simulink model "sampleModel7125_pp"  (R2018a)
settings: Solver=VariableStepAuto  StartTime=0.0  StopTime=10.0  RelTol=1e-3
undefined symbols (not defined in the file or in its folder): DiscIntNeverNeededParam
libraries: simulink x93
(part 1 of 2)
settings Model: Creator=cyfuzz  LastModifiedBy=ishaf
settings CodeAppCC: StateflowObjectComments=on

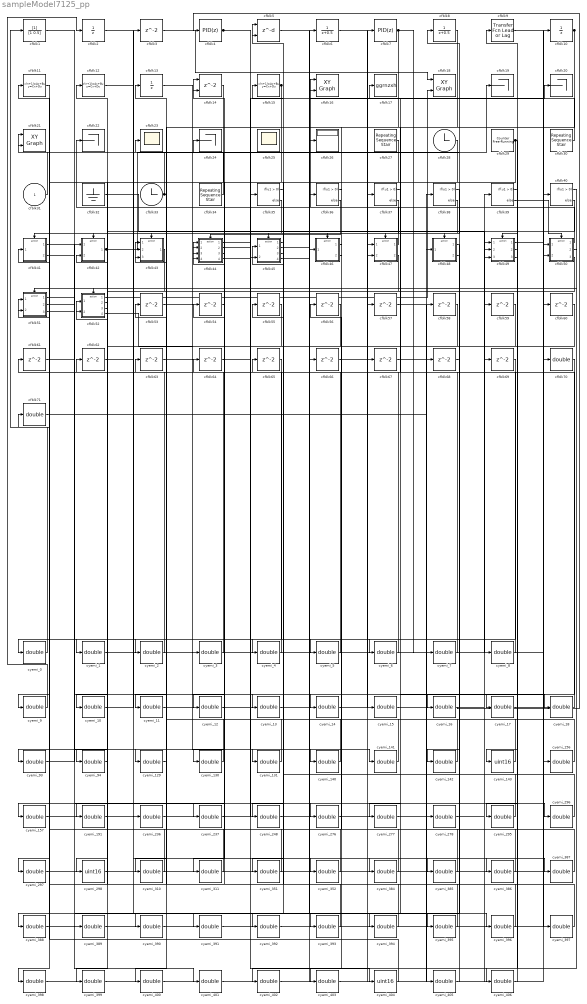
== system sampleModel7125_pp ==
  cfblk31 : Inport
  cfblk1 : DiscreteFilter  SampleTime=1
  cfblk10 : UnitDelay
  cfblk11 : DiscreteStateSpace
  cfblk12 : DiscreteStateSpace
  cfblk13 : UnitDelay
  cfblk14 : Delay  ShowEnablePort=on  SampleTime=1
      settings: InputPortMap=u0,e6
  cfblk15 : DiscreteStateSpace
  cfblk16 : simulink/Sinks/XY Graph  xmin=-1  xmax=1  ymin=-1  ymax=1  st=-1
  cfblk17 : ToWorkspace  VariableName=ggrnzxh  SaveFormat=Timeseries  SampleTime=-1
  cfblk18 : simulink/Sinks/XY Graph  xmin=-1  xmax=1  ymin=-1  ymax=1  st=-1
  cfblk{19..20,22,24} (4 alike) : Terminator
  cfblk2 : UnitDelay
  cfblk21 : simulink/Sinks/XY Graph  xmin=-1  xmax=1  ymin=-1  ymax=1  st=-1
  cfblk23 : Scope
  cfblk25 : Scope
      settings: Floating=on
  cfblk26 : Display
  cfblk27 : simulink/Sources/Repeating Sequence Stair  OutValues=[3 1 4 2 1].'  tsamp=1  OutMin=[]  OutMax=[]  OutDataTypeStr=double  OutputDataTypeScalingMode=double  OutDataType=fixdt(0,8)  ConRadixGroup=Best Precision: Vector-wise  OutScaling=2^-12
  cfblk28 : Clock
  cfblk29 : simulink/Sources/Counter Free-Running  NumBits=16  tsamp=1
  cfblk{3,53..69} (18 alike) : Delay  SampleTime=1
  cfblk30 : simulink/Sources/Repeating Sequence Stair  OutValues=[3 1 4 2 1].'  tsamp=1  OutMin=[]  OutMax=[]  OutDataTypeStr=double  OutputDataTypeScalingMode=double  OutDataType=fixdt(0,8)  ConRadixGroup=Best Precision: Vector-wise  OutScaling=2^-12
  cfblk32 : Ground
  cfblk33 : Clock
  cfblk34 : simulink/Sources/Repeating Sequence Stair  OutValues=[3 1 4 2 1].'  tsamp=1  OutMin=[]  OutMax=[]  OutDataTypeStr=double  OutputDataTypeScalingMode=double  OutDataType=fixdt(0,8)  ConRadixGroup=Best Precision: Vector-wise  OutScaling=2^-12
  cfblk{35..40} (6 alike) : If  SampleTime=1
  cfblk4 : simulink/Continuous/PID Controller  Controller=PID  TimeDomain=Discrete-time  SampleTime=1  IntegratorMethod=Forward Euler  FilterMethod=Forward Euler  Form=Parallel  UseFilter=on  ControllerParametersSource=internal  P=1  I=1  D=0  N=100  InitialConditionSource=internal  InitialConditionForIntegrator=0  InitialConditionForFilter=0  ExternalReset=none  LimitOutput=off  UpperSaturationLimit=inf  LowerSaturationLimit=-inf  LinearizeAsGain=off  AntiWindupMode=none  Kb=1  TrackingMode=off  Kt=1  PParamMin=[]  PParamMax=[]  IParamMin=[]  IParamMax=[]  DParamMin=[]  DParamMax=[]  NParamMin=[]  NParamMax=[]  KbParamMin=[]  KbParamMax=[]  KtParamMin=[]  KtParamMax=[]  POutMin=[]  POutMax=[]  IOutMin=[]  IOutMax=[]  DOutMin=[]  DOutMax=[]  NOutMin=[]  NOutMax=[]  KbOutMin=[]  KbOutMax=[]  KtOutMin=[]  KtOutMax=[]  IntegratorOutMin=[]  IntegratorOutMax=[]  FilterOutMin=[]  FilterOutMax=[]  SumOutMin=[]  SumOutMax=[]  SumI1OutMin=[]  SumI1OutMax=[]  SumI2OutMin=[]  SumI2OutMax=[]  SumI3OutMin=[]  SumI3OutMax=[]  SumDOutMin=[]  SumDOutMax=[]  SaturationOutMin=[]  SaturationOutMax=[]  IntegratorContinuousStateAttributes=''  IntegratorStateMustResolveToSignalObject=off  IntegratorRTWStateStorageClass=Auto  FilterContinuousStateAttributes=''  FilterStateMustResolveToSignalObject=off  FilterRTWStateStorageClass=Auto  DifferentiatorICPrevScaledInput=0  DifferentiatorOutMin=[]  DifferentiatorOutMax=[]  FilterDiffOutCoefMin=[]  FilterDiffOutCoefMax=[]  SumDenOutMin=[]  SumDenOutMax=[]  SumNumOutMin=[]  SumNumOutMax=[]  ReciprocalOutMin=[]  ReciprocalOutMax=[]  DivideOutMin=[]  DivideOutMax=[]  TunerSelectOption=Transfer Function Based (PID Tuner App)
  cfblk41 : Subsystem  TreatAsAtomicUnit=on
  cfblk42 : Subsystem  TreatAsAtomicUnit=on
  cfblk43 : Subsystem  TreatAsAtomicUnit=on
  cfblk44 : Subsystem  TreatAsAtomicUnit=on
  cfblk45 : Subsystem  TreatAsAtomicUnit=on
  cfblk46 : Subsystem  TreatAsAtomicUnit=on
  cfblk47 : Subsystem  TreatAsAtomicUnit=on
  cfblk48 : Subsystem  TreatAsAtomicUnit=on
  cfblk49 : Subsystem  TreatAsAtomicUnit=on
  cfblk5 : Delay  DelayLengthSource=Input port  SampleTime=1
      settings: InputPortMap=u0,p1
  cfblk50 : Subsystem  TreatAsAtomicUnit=on
  cfblk51 : Subsystem  TreatAsAtomicUnit=on
  cfblk52 : Subsystem  TreatAsAtomicUnit=on
  cfblk6 : DiscreteTransferFcn  SampleTime=1
  cfblk7 : simulink/Continuous/PID Controller  Controller=PID  TimeDomain=Discrete-time  SampleTime=1  IntegratorMethod=Forward Euler  FilterMethod=Forward Euler  Form=Parallel  UseFilter=on  ControllerParametersSource=internal  P=1  I=1  D=0  N=100  InitialConditionSource=internal  InitialConditionForIntegrator=0  InitialConditionForFilter=0  ExternalReset=none  LimitOutput=off  UpperSaturationLimit=inf  LowerSaturationLimit=-inf  LinearizeAsGain=off  AntiWindupMode=none  Kb=1  TrackingMode=off  Kt=1  PParamMin=[]  PParamMax=[]  IParamMin=[]  IParamMax=[]  DParamMin=[]  DParamMax=[]  NParamMin=[]  NParamMax=[]  KbParamMin=[]  KbParamMax=[]  KtParamMin=[]  KtParamMax=[]  POutMin=[]  POutMax=[]  IOutMin=[]  IOutMax=[]  DOutMin=[]  DOutMax=[]  NOutMin=[]  NOutMax=[]  KbOutMin=[]  KbOutMax=[]  KtOutMin=[]  KtOutMax=[]  IntegratorOutMin=[]  IntegratorOutMax=[]  FilterOutMin=[]  FilterOutMax=[]  SumOutMin=[]  SumOutMax=[]  SumI1OutMin=[]  SumI1OutMax=[]  SumI2OutMin=[]  SumI2OutMax=[]  SumI3OutMin=[]  SumI3OutMax=[]  SumDOutMin=[]  SumDOutMax=[]  SaturationOutMin=[]  SaturationOutMax=[]  IntegratorContinuousStateAttributes=''  IntegratorStateMustResolveToSignalObject=off  IntegratorRTWStateStorageClass=Auto  FilterContinuousStateAttributes=''  FilterStateMustResolveToSignalObject=off  FilterRTWStateStorageClass=Auto  DifferentiatorICPrevScaledInput=0  DifferentiatorOutMin=[]  DifferentiatorOutMax=[]  FilterDiffOutCoefMin=[]  FilterDiffOutCoefMax=[]  SumDenOutMin=[]  SumDenOutMax=[]  SumNumOutMin=[]  SumNumOutMax=[]  ReciprocalOutMin=[]  ReciprocalOutMax=[]  DivideOutMin=[]  DivideOutMax=[]  TunerSelectOption=Transfer Function Based (PID Tuner App)
  cfblk70 : DataTypeConversion  OutDataTypeStr=double
  cfblk71 : DataTypeConversion  OutDataTypeStr=double
  cfblk8 : DiscreteTransferFcn  SampleTime=1
  cfblk9 : simulink/Discrete/Transfer Fcn Lead or Lag  PoleZ=0.95  ZeroZ=0.75  ICPrevOutput=0.0  ICPrevInput=0.0  DoSatur=off
      settings: SourceProductName=Simulink  SourceProductBaseCode=SL
  cyemi_{0..18,93..94,129..131,140..142,156..157,191,236..237,248,276..278,295..297,310..311,351..352,384..403,405..406} (65 alike) : DataTypeConversion  OutDataTypeStr=double
  cyemi_143 : DataTypeConversion  OutDataTypeStr=uint16
  cyemi_298 : DataTypeConversion  OutDataTypeStr=uint16
  cyemi_404 : DataTypeConversion  OutDataTypeStr=uint16
  wires:
  cfblk34/1 -> cfblk24/1
  cfblk3/1 -> cfblk18/1
  cfblk15/1 -> cyemi_398/1, cyemi_399/1
  cfblk47/1(cfblk2) -> cfblk16/1
  cfblk30/1 -> cfblk16/2
  cfblk7/1 -> cyemi_7/1, cyemi_400/1
  cfblk33/1 -> cfblk21/2, cyemi_2/1
  cfblk31/1 -> cfblk21/1
  cfblk29/1 -> cyemi_143/1, cyemi_298/1
  cfblk52/1(cfblk2) -> cfblk18/2
  cfblk10/1 -> cyemi_5/1, cyemi_394/1
  cfblk48/2(cfblk7) -> cfblk23/1
  cfblk42/1(cfblk2) -> cfblk19/1, cyemi_384/1
  cfblk50/1(cfblk2) -> cfblk22/1
  cfblk4/1 -> cyemi_385/1, cyemi_386/1
  cfblk45/4(cfblk16) -> cfblk26/1
  cfblk44/2(cfblk15) -> cfblk20/1
  cfblk35/1 -> cfblk41/Action
  cfblk35/2 -> cfblk42/Action
  cfblk36/1 -> cfblk43/Action
  cfblk36/2 -> cfblk44/Action
  cfblk37/1 -> cfblk45/Action
  cfblk37/2 -> cfblk46/Action
  cfblk38/1 -> cfblk47/Action
  cfblk38/2 -> cfblk48/Action
  cfblk39/1 -> cfblk49/Action
  cfblk39/2 -> cfblk50/Action
  cfblk40/1 -> cfblk51/Action
  cfblk40/2 -> cfblk52/Action
  cyemi_0/1 -> cfblk1/1
  cfblk11/1 -> cyemi_0/1
  cyemi_1/1 -> cfblk10/1
  cfblk52/2(cfblk8) -> cyemi_1/1
  cyemi_2/1 -> cfblk11/1
  cyemi_3/1 -> cfblk12/1
  cfblk52/4(cfblk10) -> cyemi_3/1
  cyemi_4/1 -> cfblk13/1
  cfblk45/3(cfblk15) -> cyemi_4/1
  cyemi_5/1 -> cfblk14/1
  cyemi_6/1 -> cfblk14/2
  cfblk58/1 -> cyemi_6/1
  cyemi_7/1 -> cfblk15/1
  cyemi_8/1 -> cfblk17/1
  cfblk32/1 -> cyemi_8/1
  cyemi_9/1 -> cfblk2/1
  cfblk69/1 -> cyemi_9/1
  cyemi_10/1 -> cfblk3/1
  cfblk52/3(cfblk9) -> cyemi_10/1
  cyemi_11/1 -> cfblk35/1
  cfblk14/1 -> cyemi_11/1
  cyemi_12/1 -> cfblk36/1
  cfblk28/1 -> cyemi_12/1
  cyemi_13/1 -> cfblk37/1
  cfblk51/3(cfblk16) -> cyemi_13/1
  cyemi_14/1 -> cfblk38/1
  cfblk64/1 -> cyemi_14/1
  cyemi_15/1 -> cfblk39/1
  cfblk66/1 -> cyemi_15/1
  cyemi_16/1 -> cfblk4/1
  cfblk6/1 -> cyemi_16/1
  cyemi_17/1 -> cfblk40/1
  cfblk57/1 -> cyemi_17/1
  cyemi_18/1 -> cfblk41/1(cfblk1)
  cfblk13/1 -> cyemi_18/1
  cyemi_93/1 -> cfblk42/1(cfblk1)
  cfblk50/3(cfblk14) -> cyemi_93/1
  cyemi_94/1 -> cfblk42/2(cfblk13)
  cfblk43/1(cfblk2) -> cyemi_94/1
  cyemi_129/1 -> cfblk43/1(cfblk1)
  cfblk1/1 -> cyemi_129/1
  cyemi_130/1 -> cfblk43/2(cfblk8)
  cfblk54/1 -> cyemi_130/1
  cyemi_131/1 -> cfblk43/3(cfblk9)
  cfblk53/1 -> cyemi_131/1
  cyemi_140/1 -> cfblk44/1(cfblk1)
  cfblk51/1(cfblk2) -> cyemi_140/1
  cyemi_141/1 -> cfblk44/2(cfblk12)
  cfblk63/1 -> cyemi_141/1
  cyemi_142/1 -> cfblk44/3(cfblk13)
  cfblk68/1 -> cyemi_142/1
  cyemi_143/1 -> cfblk44/4(cfblk14)
  cyemi_156/1 -> cfblk45/1(cfblk1)
  cfblk49/1(cfblk2) -> cyemi_156/1
  cyemi_157/1 -> cfblk45/2(cfblk13)
  cfblk44/3(cfblk16) -> cyemi_157/1
  cyemi_191/1 -> cfblk46/1(cfblk1)
  cfblk59/1 -> cyemi_191/1
  cyemi_236/1 -> cfblk47/1(cfblk1)
  cfblk2/1 -> cyemi_236/1
  cyemi_237/1 -> cfblk47/2(cfblk12)
  cfblk55/1 -> cyemi_237/1
  cyemi_248/1 -> cfblk48/1(cfblk1)
  cfblk56/1 -> cyemi_248/1
  cyemi_276/1 -> cfblk49/1(cfblk1)
  cfblk61/1 -> cyemi_276/1
  cyemi_277/1 -> cfblk49/2(cfblk14)
  cfblk70/1 -> cyemi_277/1
  cyemi_278/1 -> cfblk49/3(cfblk15)
  cfblk67/1 -> cyemi_278/1
  cyemi_295/1 -> cfblk5/1
  cfblk49/2(cfblk16) -> cyemi_295/1
  cyemi_296/1 -> cfblk5/2
  cfblk44/4(cfblk17) -> cyemi_296/1
  cyemi_297/1 -> cfblk50/1(cfblk1)
  cfblk65/1 -> cyemi_297/1
  cyemi_298/1 -> cfblk50/2(cfblk12)
  cyemi_310/1 -> cfblk51/1(cfblk1)
  cfblk47/2(cfblk13) -> cyemi_310/1
  cyemi_311/1 -> cfblk51/2(cfblk14)
  cfblk60/1 -> cyemi_311/1
  cyemi_351/1 -> cfblk52/1(cfblk1)
  cfblk27/1 -> cyemi_351/1
  cyemi_352/1 -> cfblk52/2(cfblk7)
  cfblk62/1 -> cyemi_352/1
  cyemi_384/1 -> cfblk53/1
  cyemi_385/1 -> cfblk54/1
  cyemi_386/1 -> cfblk55/1
  cyemi_387/1 -> cfblk56/1
  cfblk45/2(cfblk14) -> cyemi_387/1
  cyemi_388/1 -> cfblk57/1
  cfblk48/1(cfblk2) -> cyemi_388/1
  cyemi_389/1 -> cfblk58/1
  cfblk41/1(cfblk2) -> cyemi_389/1
  cyemi_390/1 -> cfblk59/1
  cfblk41/2(cfblk14) -> cyemi_390/1
  cyemi_391/1 -> cfblk6/1
  cfblk45/1(cfblk2) -> cyemi_391/1
  cyemi_392/1 -> cfblk60/1
  cfblk46/1(cfblk2) -> cyemi_392/1
  cyemi_393/1 -> cfblk61/1
  cfblk46/2(cfblk16) -> cyemi_393/1
  cyemi_394/1 -> cfblk62/1
  cyemi_395/1 -> cfblk63/1
  cfblk12/1 -> cyemi_395/1
  cyemi_396/1 -> cfblk64/1
  cfblk5/1 -> cyemi_396/1
  cyemi_397/1 -> cfblk65/1
  cfblk9/1 -> cyemi_397/1
  cyemi_398/1 -> cfblk66/1
  cyemi_399/1 -> cfblk67/1
  cyemi_400/1 -> cfblk68/1
  cyemi_401/1 -> cfblk69/1
  cfblk51/2(cfblk15) -> cyemi_401/1
  cyemi_402/1 -> cfblk7/1
  cfblk50/2(cfblk13) -> cyemi_402/1
  cyemi_403/1 -> cfblk70/1
  cfblk8/1 -> cyemi_403/1
  cyemi_404/1 -> cfblk71/1
  cfblk44/1(cfblk2) -> cyemi_404/1
  cyemi_405/1 -> cfblk8/1
  cfblk71/1 -> cyemi_405/1
  cyemi_406/1 -> cfblk9/1
  cfblk49/3(cfblk17) -> cyemi_406/1

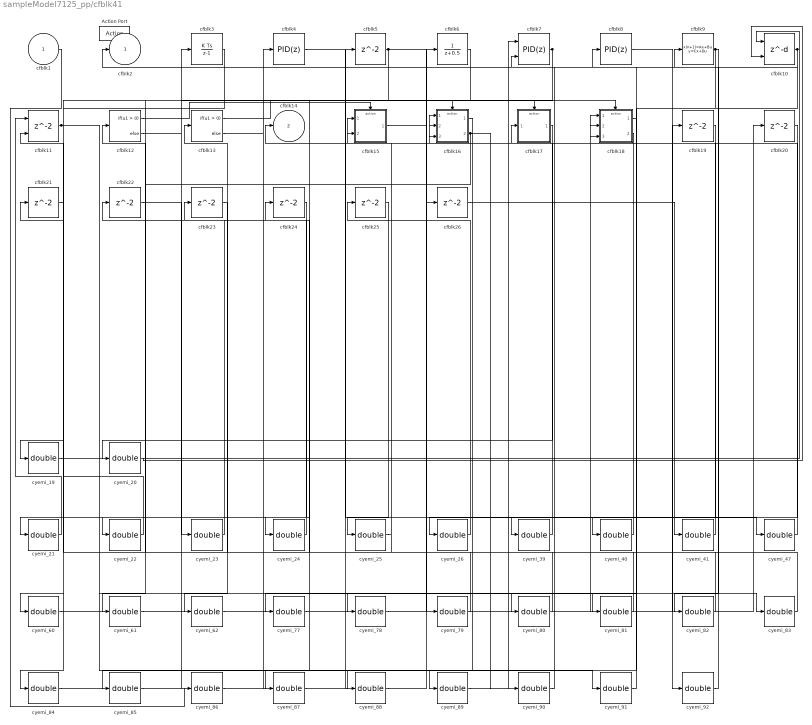
== system sampleModel7125_pp/cfblk41 ==
  cfblk1 : Inport
  Action Port : ActionPort  ActionType=then
  cfblk10 : Delay  DelayLengthSource=Input port
      settings: InputPortMap=u0,p1
  cfblk11 : Delay  ShowEnablePort=on
      settings: InputPortMap=u0,e6
  cfblk12 : If  SampleTime=1
  cfblk13 : If  SampleTime=1
  cfblk15 : Subsystem  TreatAsAtomicUnit=on
  cfblk16 : Subsystem  TreatAsAtomicUnit=on
  cfblk17 : Subsystem  TreatAsAtomicUnit=on
  cfblk18 : Subsystem  TreatAsAtomicUnit=on
  cfblk{5,19..26} (9 alike) : Delay
  cfblk3 : DiscreteIntegrator  SampleTime=-1  OutDataTypeStr=double  ICPrevOutput=DiscIntNeverNeededParam  ICPrevScaledInput=DiscIntNeverNeededParam
  cfblk4 : simulink/Continuous/PID Controller  Controller=PID  TimeDomain=Discrete-time  SampleTime=-1  IntegratorMethod=Forward Euler  FilterMethod=Forward Euler  Form=Parallel  UseFilter=on  ControllerParametersSource=internal  P=1  I=1  D=0  N=100  InitialConditionSource=internal  InitialConditionForIntegrator=0  InitialConditionForFilter=0  ExternalReset=none  LimitOutput=off  UpperSaturationLimit=inf  LowerSaturationLimit=-inf  LinearizeAsGain=off  AntiWindupMode=none  Kb=1  TrackingMode=off  Kt=1  PParamMin=[]  PParamMax=[]  IParamMin=[]  IParamMax=[]  DParamMin=[]  DParamMax=[]  NParamMin=[]  NParamMax=[]  KbParamMin=[]  KbParamMax=[]  KtParamMin=[]  KtParamMax=[]  POutMin=[]  POutMax=[]  IOutMin=[]  IOutMax=[]  DOutMin=[]  DOutMax=[]  NOutMin=[]  NOutMax=[]  KbOutMin=[]  KbOutMax=[]  KtOutMin=[]  KtOutMax=[]  IntegratorOutMin=[]  IntegratorOutMax=[]  FilterOutMin=[]  FilterOutMax=[]  SumOutMin=[]  SumOutMax=[]  SumI1OutMin=[]  SumI1OutMax=[]  SumI2OutMin=[]  SumI2OutMax=[]  SumI3OutMin=[]  SumI3OutMax=[]  SumDOutMin=[]  SumDOutMax=[]  SaturationOutMin=[]  SaturationOutMax=[]  IntegratorContinuousStateAttributes=''  IntegratorStateMustResolveToSignalObject=off  IntegratorRTWStateStorageClass=Auto  FilterContinuousStateAttributes=''  FilterStateMustResolveToSignalObject=off  FilterRTWStateStorageClass=Auto  DifferentiatorICPrevScaledInput=0  DifferentiatorOutMin=[]  DifferentiatorOutMax=[]  FilterDiffOutCoefMin=[]  FilterDiffOutCoefMax=[]  SumDenOutMin=[]  SumDenOutMax=[]  SumNumOutMin=[]  SumNumOutMax=[]  ReciprocalOutMin=[]  ReciprocalOutMax=[]  DivideOutMin=[]  DivideOutMax=[]  TunerSelectOption=Transfer Function Based (PID Tuner App)
  cfblk6 : DiscreteTransferFcn
  cfblk7 : simulink/Continuous/PID Controller (2DOF)  Controller=PID  TimeDomain=Discrete-time  SampleTime=-1  IntegratorMethod=Forward Euler  FilterMethod=Forward Euler  Form=Parallel  UseFilter=on  ControllerParametersSource=internal  P=1  I=1  D=0  N=100  b=1  c=1  InitialConditionSource=internal  InitialConditionForIntegrator=0  InitialConditionForFilter=0  ExternalReset=none  LimitOutput=off  UpperSaturationLimit=inf  LowerSaturationLimit=-inf  LinearizeAsGain=off  AntiWindupMode=none  Kb=1  TrackingMode=off  Kt=1  PParamMin=[]  PParamMax=[]  IParamMin=[]  IParamMax=[]  DParamMin=[]  DParamMax=[]  NParamMin=[]  NParamMax=[]  bParamMin=[]  bParamMax=[]  cParamMin=[]  cParamMax=[]  KbParamMin=[]  KbParamMax=[]  KtParamMin=[]  KtParamMax=[]  POutMin=[]  POutMax=[]  IOutMin=[]  IOutMax=[]  DOutMin=[]  DOutMax=[]  NOutMin=[]  NOutMax=[]  bOutMin=[]  bOutMax=[]  cOutMin=[]  cOutMax=[]  KbOutMin=[]  KbOutMax=[]  KtOutMin=[]  KtOutMax=[]  IntegratorOutMin=[]  IntegratorOutMax=[]  FilterOutMin=[]  FilterOutMax=[]  SumOutMin=[]  SumOutMax=[]  Sum1OutMin=[]  Sum1OutMax=[]  Sum2OutMin=[]  Sum2OutMax=[]  Sum3OutMin=[]  Sum3OutMax=[]  SumI1OutMin=[]  SumI1OutMax=[]  SumI2OutMin=[]  SumI2OutMax=[]  SumI3OutMin=[]  SumI3OutMax=[]  SumDOutMin=[]  SumDOutMax=[]  SaturationOutMin=[]  SaturationOutMax=[]  IntegratorContinuousStateAttributes=''  IntegratorStateMustResolveToSignalObject=off  IntegratorRTWStateStorageClass=Auto  FilterContinuousStateAttributes=''  FilterStateMustResolveToSignalObject=off  FilterRTWStateStorageClass=Auto  DifferentiatorICPrevScaledInput=0  DifferentiatorOutMin=[]  DifferentiatorOutMax=[]  FilterDiffOutCoefMin=[]  FilterDiffOutCoefMax=[]  SumDenOutMin=[]  SumDenOutMax=[]  SumNumOutMin=[]  SumNumOutMax=[]  ReciprocalOutMin=[]  ReciprocalOutMax=[]  DivideOutMin=[]  DivideOutMax=[]  TunerSelectOption=Transfer Function Based (PID Tuner App)
  cfblk8 : simulink/Continuous/PID Controller  Controller=PID  TimeDomain=Discrete-time  SampleTime=-1  IntegratorMethod=Forward Euler  FilterMethod=Forward Euler  Form=Parallel  UseFilter=on  ControllerParametersSource=internal  P=1  I=1  D=0  N=100  InitialConditionSource=internal  InitialConditionForIntegrator=0  InitialConditionForFilter=0  ExternalReset=none  LimitOutput=off  UpperSaturationLimit=inf  LowerSaturationLimit=-inf  LinearizeAsGain=off  AntiWindupMode=none  Kb=1  TrackingMode=off  Kt=1  PParamMin=[]  PParamMax=[]  IParamMin=[]  IParamMax=[]  DParamMin=[]  DParamMax=[]  NParamMin=[]  NParamMax=[]  KbParamMin=[]  KbParamMax=[]  KtParamMin=[]  KtParamMax=[]  POutMin=[]  POutMax=[]  IOutMin=[]  IOutMax=[]  DOutMin=[]  DOutMax=[]  NOutMin=[]  NOutMax=[]  KbOutMin=[]  KbOutMax=[]  KtOutMin=[]  KtOutMax=[]  IntegratorOutMin=[]  IntegratorOutMax=[]  FilterOutMin=[]  FilterOutMax=[]  SumOutMin=[]  SumOutMax=[]  SumI1OutMin=[]  SumI1OutMax=[]  SumI2OutMin=[]  SumI2OutMax=[]  SumI3OutMin=[]  SumI3OutMax=[]  SumDOutMin=[]  SumDOutMax=[]  SaturationOutMin=[]  SaturationOutMax=[]  IntegratorContinuousStateAttributes=''  IntegratorStateMustResolveToSignalObject=off  IntegratorRTWStateStorageClass=Auto  FilterContinuousStateAttributes=''  FilterStateMustResolveToSignalObject=off  FilterRTWStateStorageClass=Auto  DifferentiatorICPrevScaledInput=0  DifferentiatorOutMin=[]  DifferentiatorOutMax=[]  FilterDiffOutCoefMin=[]  FilterDiffOutCoefMax=[]  SumDenOutMin=[]  SumDenOutMax=[]  SumNumOutMin=[]  SumNumOutMax=[]  ReciprocalOutMin=[]  ReciprocalOutMax=[]  DivideOutMin=[]  DivideOutMax=[]  TunerSelectOption=Transfer Function Based (PID Tuner App)
  cfblk9 : DiscreteStateSpace  SampleTime=-1
  cyemi_{19..26,39..41,47,60..62,77..92} (31 alike) : DataTypeConversion  OutDataTypeStr=double
  cfblk2 : Outport
  cfblk14 : Outport  Port=2
  wires:
  cfblk7/1 -> cyemi_84/1, cyemi_87/1
  cfblk9/1 -> cyemi_82/1, cyemi_85/1
  cfblk10/1 -> cfblk2/1, cyemi_77/1, cyemi_78/1, cyemi_81/1
  cfblk16/2(cfblk9) -> cyemi_61/1, cyemi_89/1, cyemi_90/1
  cfblk5/1 -> cyemi_22/1, cyemi_47/1
  cfblk11/1 -> cyemi_83/1, cyemi_91/1
  cfblk18/2(cfblk17) -> cfblk14/1
  cfblk12/1 -> cfblk15/Action
  cfblk12/2 -> cfblk16/Action
  cfblk13/1 -> cfblk17/Action
  cfblk13/2 -> cfblk18/Action
  cyemi_19/1 -> cfblk10/1
  cfblk3/1 -> cyemi_19/1
  cyemi_20/1 -> cfblk10/2
  cfblk17/1(cfblk2) -> cyemi_20/1
  cyemi_21/1 -> cfblk11/1
  cfblk24/1 -> cyemi_21/1
  cyemi_22/1 -> cfblk11/2
  cyemi_23/1 -> cfblk12/1
  cfblk22/1 -> cyemi_23/1
  cyemi_24/1 -> cfblk13/1
  cfblk6/1 -> cyemi_24/1
  cyemi_25/1 -> cfblk15/1(cfblk1)
  cfblk25/1 -> cyemi_25/1
  cyemi_26/1 -> cfblk15/2(cfblk10)
  cfblk20/1 -> cyemi_26/1
  cyemi_39/1 -> cfblk16/1(cfblk1)
  cfblk19/1 -> cyemi_39/1
  cyemi_40/1 -> cfblk16/2(cfblk7)
  cfblk4/1 -> cyemi_40/1
  cyemi_41/1 -> cfblk16/3(cfblk8)
  cfblk26/1 -> cyemi_41/1
  cyemi_47/1 -> cfblk17/1(cfblk1)
  cyemi_60/1 -> cfblk18/1(cfblk1)
  cfblk21/1 -> cyemi_60/1
  cyemi_61/1 -> cfblk18/2(cfblk15)
  cyemi_62/1 -> cfblk18/3(cfblk16)
  cfblk23/1 -> cyemi_62/1
  cyemi_77/1 -> cfblk19/1
  cyemi_78/1 -> cfblk20/1
  cyemi_79/1 -> cfblk21/1
  cfblk15/1(cfblk2) -> cyemi_79/1
  cyemi_80/1 -> cfblk22/1
  cfblk18/1(cfblk2) -> cyemi_80/1
  cyemi_81/1 -> cfblk23/1
  cyemi_82/1 -> cfblk24/1
  cyemi_83/1 -> cfblk25/1
  cyemi_84/1 -> cfblk26/1
  cyemi_85/1 -> cfblk3/1
  cyemi_86/1 -> cfblk4/1
  cfblk1/1 -> cyemi_86/1
  cyemi_87/1 -> cfblk5/1
  cyemi_88/1 -> cfblk6/1
  cfblk16/1(cfblk2) -> cyemi_88/1
  cyemi_89/1 -> cfblk7/1
  cyemi_90/1 -> cfblk7/2
  cyemi_91/1 -> cfblk8/1
  cyemi_92/1 -> cfblk9/1
  cfblk8/1 -> cyemi_92/1

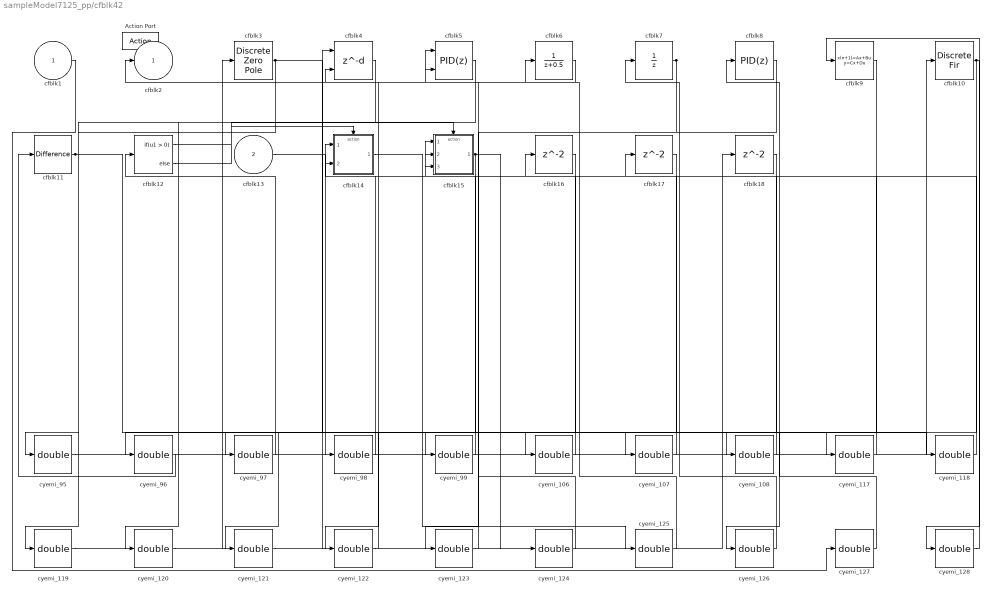
== system sampleModel7125_pp/cfblk42 ==
  cfblk1 : Inport
  cfblk13 : Inport  Port=2
  Action Port : ActionPort  ActionType=else
  cfblk10 : DiscreteFir
  cfblk11 : simulink/Discrete/Difference  ICPrevInput=0.0  OutMin=[]  OutMax=[]  OutDataTypeStr=double  OutputDataTypeScalingMode=double  OutDataType=fixdt(1, 16)  OutScaling=2^-10  DoSatur=off
  cfblk12 : If  SampleTime=1
  cfblk14 : Subsystem  TreatAsAtomicUnit=on
  cfblk15 : Subsystem  TreatAsAtomicUnit=on
  cfblk16 : Delay
  cfblk17 : Delay
  cfblk18 : Delay
  cfblk3 : DiscreteZeroPole  Poles=[0 0.5]  Gain=1  SampleTime=-1
  cfblk4 : Delay  DelayLengthSource=Input port
      settings: InputPortMap=u0,p1
  cfblk5 : simulink/Continuous/PID Controller (2DOF)  Controller=PID  TimeDomain=Discrete-time  SampleTime=-1  IntegratorMethod=Forward Euler  FilterMethod=Forward Euler  Form=Parallel  UseFilter=on  ControllerParametersSource=internal  P=1  I=1  D=0  N=100  b=1  c=1  InitialConditionSource=internal  InitialConditionForIntegrator=0  InitialConditionForFilter=0  ExternalReset=none  LimitOutput=off  UpperSaturationLimit=inf  LowerSaturationLimit=-inf  LinearizeAsGain=off  AntiWindupMode=none  Kb=1  TrackingMode=off  Kt=1  PParamMin=[]  PParamMax=[]  IParamMin=[]  IParamMax=[]  DParamMin=[]  DParamMax=[]  NParamMin=[]  NParamMax=[]  bParamMin=[]  bParamMax=[]  cParamMin=[]  cParamMax=[]  KbParamMin=[]  KbParamMax=[]  KtParamMin=[]  KtParamMax=[]  POutMin=[]  POutMax=[]  IOutMin=[]  IOutMax=[]  DOutMin=[]  DOutMax=[]  NOutMin=[]  NOutMax=[]  bOutMin=[]  bOutMax=[]  cOutMin=[]  cOutMax=[]  KbOutMin=[]  KbOutMax=[]  KtOutMin=[]  KtOutMax=[]  IntegratorOutMin=[]  IntegratorOutMax=[]  FilterOutMin=[]  FilterOutMax=[]  SumOutMin=[]  SumOutMax=[]  Sum1OutMin=[]  Sum1OutMax=[]  Sum2OutMin=[]  Sum2OutMax=[]  Sum3OutMin=[]  Sum3OutMax=[]  SumI1OutMin=[]  SumI1OutMax=[]  SumI2OutMin=[]  SumI2OutMax=[]  SumI3OutMin=[]  SumI3OutMax=[]  SumDOutMin=[]  SumDOutMax=[]  SaturationOutMin=[]  SaturationOutMax=[]  IntegratorContinuousStateAttributes=''  IntegratorStateMustResolveToSignalObject=off  IntegratorRTWStateStorageClass=Auto  FilterContinuousStateAttributes=''  FilterStateMustResolveToSignalObject=off  FilterRTWStateStorageClass=Auto  DifferentiatorICPrevScaledInput=0  DifferentiatorOutMin=[]  DifferentiatorOutMax=[]  FilterDiffOutCoefMin=[]  FilterDiffOutCoefMax=[]  SumDenOutMin=[]  SumDenOutMax=[]  SumNumOutMin=[]  SumNumOutMax=[]  ReciprocalOutMin=[]  ReciprocalOutMax=[]  DivideOutMin=[]  DivideOutMax=[]  TunerSelectOption=Transfer Function Based (PID Tuner App)
  cfblk6 : DiscreteTransferFcn
  cfblk7 : UnitDelay  SampleTime=-1
  cfblk8 : simulink/Continuous/PID Controller  Controller=PID  TimeDomain=Discrete-time  SampleTime=-1  IntegratorMethod=Forward Euler  FilterMethod=Forward Euler  Form=Parallel  UseFilter=on  ControllerParametersSource=internal  P=1  I=1  D=0  N=100  InitialConditionSource=internal  InitialConditionForIntegrator=0  InitialConditionForFilter=0  ExternalReset=none  LimitOutput=off  UpperSaturationLimit=inf  LowerSaturationLimit=-inf  LinearizeAsGain=off  AntiWindupMode=none  Kb=1  TrackingMode=off  Kt=1  PParamMin=[]  PParamMax=[]  IParamMin=[]  IParamMax=[]  DParamMin=[]  DParamMax=[]  NParamMin=[]  NParamMax=[]  KbParamMin=[]  KbParamMax=[]  KtParamMin=[]  KtParamMax=[]  POutMin=[]  POutMax=[]  IOutMin=[]  IOutMax=[]  DOutMin=[]  DOutMax=[]  NOutMin=[]  NOutMax=[]  KbOutMin=[]  KbOutMax=[]  KtOutMin=[]  KtOutMax=[]  IntegratorOutMin=[]  IntegratorOutMax=[]  FilterOutMin=[]  FilterOutMax=[]  SumOutMin=[]  SumOutMax=[]  SumI1OutMin=[]  SumI1OutMax=[]  SumI2OutMin=[]  SumI2OutMax=[]  SumI3OutMin=[]  SumI3OutMax=[]  SumDOutMin=[]  SumDOutMax=[]  SaturationOutMin=[]  SaturationOutMax=[]  IntegratorContinuousStateAttributes=''  IntegratorStateMustResolveToSignalObject=off  IntegratorRTWStateStorageClass=Auto  FilterContinuousStateAttributes=''  FilterStateMustResolveToSignalObject=off  FilterRTWStateStorageClass=Auto  DifferentiatorICPrevScaledInput=0  DifferentiatorOutMin=[]  DifferentiatorOutMax=[]  FilterDiffOutCoefMin=[]  FilterDiffOutCoefMax=[]  SumDenOutMin=[]  SumDenOutMax=[]  SumNumOutMin=[]  SumNumOutMax=[]  ReciprocalOutMin=[]  ReciprocalOutMax=[]  DivideOutMin=[]  DivideOutMax=[]  TunerSelectOption=Transfer Function Based (PID Tuner App)
  cfblk9 : DiscreteStateSpace  SampleTime=-1
  cyemi_{95..99,106..108,117..128} (20 alike) : DataTypeConversion  OutDataTypeStr=double
  cfblk2 : Outport
  wires:
  cfblk10/1 -> cyemi_126/1, cyemi_128/1
  cfblk11/1 -> cyemi_117/1, cyemi_118/1
  cfblk6/1 -> cfblk2/1
  cfblk7/1 -> cyemi_97/1, cyemi_123/1
  cfblk3/1 -> cyemi_95/1, cyemi_108/1
  cfblk15/1(cfblk2) -> cyemi_122/1, cyemi_124/1
  cfblk12/1 -> cfblk14/Action
  cfblk12/2 -> cfblk15/Action
  cyemi_95/1 -> cfblk10/1
  cyemi_96/1 -> cfblk11/1
  cfblk4/1 -> cyemi_96/1
  cyemi_97/1 -> cfblk12/1
  cyemi_98/1 -> cfblk14/1(cfblk1)
  cfblk13/1 -> cyemi_98/1
  cyemi_99/1 -> cfblk14/2(cfblk8)
  cfblk8/1 -> cyemi_99/1
  cyemi_106/1 -> cfblk15/1(cfblk1)
  cfblk9/1 -> cyemi_106/1
  cyemi_107/1 -> cfblk15/2(cfblk11)
  cfblk18/1 -> cyemi_107/1
  cyemi_108/1 -> cfblk15/3(cfblk12)
  cyemi_117/1 -> cfblk16/1
  cyemi_118/1 -> cfblk17/1
  cyemi_119/1 -> cfblk18/1
  cfblk5/1 -> cyemi_119/1
  cyemi_120/1 -> cfblk3/1
  cfblk17/1 -> cyemi_120/1
  cyemi_121/1 -> cfblk4/1
  cfblk16/1 -> cyemi_121/1
  cyemi_122/1 -> cfblk4/2
  cyemi_123/1 -> cfblk5/1
  cyemi_124/1 -> cfblk5/2
  cyemi_125/1 -> cfblk6/1
  cfblk14/1(cfblk2) -> cyemi_125/1
  cyemi_126/1 -> cfblk7/1
  cyemi_127/1 -> cfblk8/1
  cfblk1/1 -> cyemi_127/1
  cyemi_128/1 -> cfblk9/1

== system sampleModel7125_pp/cfblk43 ==
  cfblk1 : Inport
  cfblk8 : Inport  Port=2
  cfblk9 : Inport  Port=3
  Action Port : ActionPort  ActionType=then
  cfblk10 : Delay
  cfblk3 : simulink/Continuous/PID Controller  Controller=PID  TimeDomain=Discrete-time  SampleTime=-1  IntegratorMethod=Forward Euler  FilterMethod=Forward Euler  Form=Parallel  UseFilter=on  ControllerParametersSource=internal  P=1  I=1  D=0  N=100  InitialConditionSource=internal  InitialConditionForIntegrator=0  InitialConditionForFilter=0  ExternalReset=none  LimitOutput=off  UpperSaturationLimit=inf  LowerSaturationLimit=-inf  LinearizeAsGain=off  AntiWindupMode=none  Kb=1  TrackingMode=off  Kt=1  PParamMin=[]  PParamMax=[]  IParamMin=[]  IParamMax=[]  DParamMin=[]  DParamMax=[]  NParamMin=[]  NParamMax=[]  KbParamMin=[]  KbParamMax=[]  KtParamMin=[]  KtParamMax=[]  POutMin=[]  POutMax=[]  IOutMin=[]  IOutMax=[]  DOutMin=[]  DOutMax=[]  NOutMin=[]  NOutMax=[]  KbOutMin=[]  KbOutMax=[]  KtOutMin=[]  KtOutMax=[]  IntegratorOutMin=[]  IntegratorOutMax=[]  FilterOutMin=[]  FilterOutMax=[]  SumOutMin=[]  SumOutMax=[]  SumI1OutMin=[]  SumI1OutMax=[]  SumI2OutMin=[]  SumI2OutMax=[]  SumI3OutMin=[]  SumI3OutMax=[]  SumDOutMin=[]  SumDOutMax=[]  SaturationOutMin=[]  SaturationOutMax=[]  IntegratorContinuousStateAttributes=''  IntegratorStateMustResolveToSignalObject=off  IntegratorRTWStateStorageClass=Auto  FilterContinuousStateAttributes=''  FilterStateMustResolveToSignalObject=off  FilterRTWStateStorageClass=Auto  DifferentiatorICPrevScaledInput=0  DifferentiatorOutMin=[]  DifferentiatorOutMax=[]  FilterDiffOutCoefMin=[]  FilterDiffOutCoefMax=[]  SumDenOutMin=[]  SumDenOutMax=[]  SumNumOutMin=[]  SumNumOutMax=[]  ReciprocalOutMin=[]  ReciprocalOutMax=[]  DivideOutMin=[]  DivideOutMax=[]  TunerSelectOption=Transfer Function Based (PID Tuner App)
  cfblk4 : DiscreteTransferFcn
  cfblk5 : Delay  ShowEnablePort=on
      settings: InputPortMap=u0,e6
  cfblk6 : Delay  ShowEnablePort=on
      settings: InputPortMap=u0,e6
  cfblk7 : DiscreteIntegrator  SampleTime=-1  OutDataTypeStr=double  ICPrevOutput=DiscIntNeverNeededParam  ICPrevScaledInput=DiscIntNeverNeededParam
  cyemi_{132..139} (8 alike) : DataTypeConversion  OutDataTypeStr=double
  cfblk2 : Outport
  wires:
  cfblk1/1 -> cfblk2/1
  cyemi_132/1 -> cfblk10/1
  cfblk6/1 -> cyemi_132/1
  cyemi_133/1 -> cfblk3/1
  cfblk10/1 -> cyemi_133/1
  cyemi_134/1 -> cfblk4/1
  cfblk7/1 -> cyemi_134/1
  cyemi_135/1 -> cfblk5/1
  cfblk8/1 -> cyemi_135/1
  cyemi_136/1 -> cfblk5/2
  cfblk9/1 -> cyemi_136/1
  cyemi_137/1 -> cfblk6/1
  cfblk5/1 -> cyemi_137/1
  cyemi_138/1 -> cfblk6/2
  cfblk4/1 -> cyemi_138/1
  cyemi_139/1 -> cfblk7/1
  cfblk3/1 -> cyemi_139/1

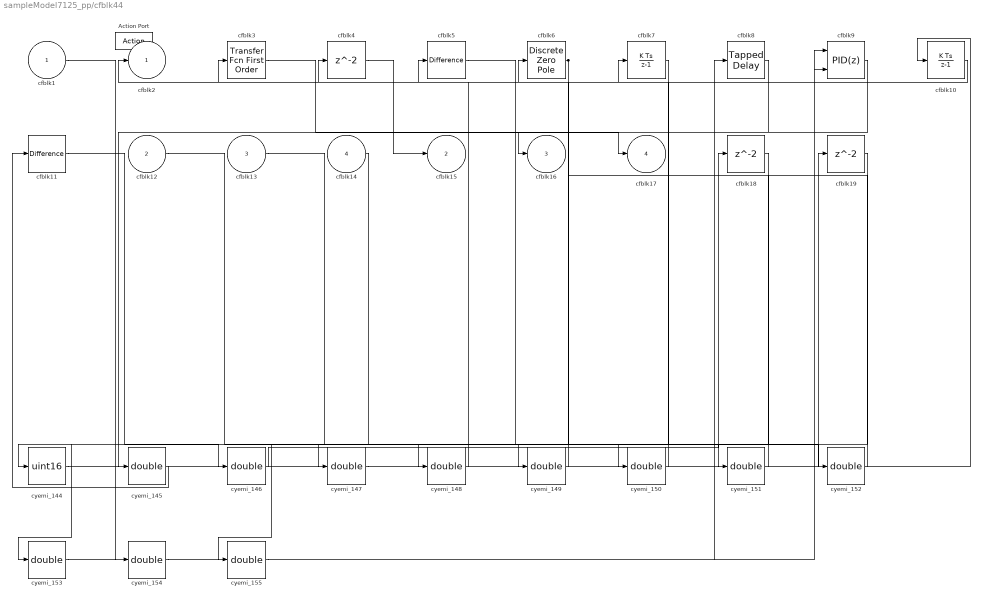
== system sampleModel7125_pp/cfblk44 ==
  cfblk1 : Inport
  cfblk12 : Inport  Port=2
  cfblk13 : Inport  Port=3
  cfblk14 : Inport  Port=4
  Action Port : ActionPort  ActionType=else
  cfblk10 : DiscreteIntegrator  SampleTime=-1  OutDataTypeStr=uint16  ICPrevOutput=DiscIntNeverNeededParam  ICPrevScaledInput=DiscIntNeverNeededParam
  cfblk11 : simulink/Discrete/Difference  ICPrevInput=0.0  OutMin=[]  OutMax=[]  OutDataTypeStr=double  OutputDataTypeScalingMode=double  OutDataType=fixdt(1, 16)  OutScaling=2^-10  DoSatur=off
  cfblk18 : Delay
  cfblk19 : Delay
  cfblk3 : simulink/Discrete/Transfer Fcn First Order  PoleZ=0.95  ICPrevOutput=0.0  DoSatur=off
      settings: SourceProductName=Simulink
  cfblk4 : Delay
  cfblk5 : simulink/Discrete/Difference  ICPrevInput=0.0  OutMin=[]  OutMax=[]  OutDataTypeStr=double  OutputDataTypeScalingMode=double  OutDataType=fixdt(1, 16)  OutScaling=2^-10  DoSatur=off
  cfblk6 : DiscreteZeroPole  Poles=[0 0.5]  Gain=1  SampleTime=-1
  cfblk7 : DiscreteIntegrator  SampleTime=-1  OutDataTypeStr=double  ICPrevOutput=DiscIntNeverNeededParam  ICPrevScaledInput=DiscIntNeverNeededParam
  cfblk8 : simulink/Discrete/Tapped Delay  vinit=0.0  samptime=-1  NumDelays=1  DelayOrder=Oldest  includeCurrent=off
  cfblk9 : simulink/Continuous/PID Controller (2DOF)  Controller=PID  TimeDomain=Discrete-time  SampleTime=-1  IntegratorMethod=Forward Euler  FilterMethod=Forward Euler  Form=Parallel  UseFilter=on  ControllerParametersSource=internal  P=1  I=1  D=0  N=100  b=1  c=1  InitialConditionSource=internal  InitialConditionForIntegrator=0  InitialConditionForFilter=0  ExternalReset=none  LimitOutput=off  UpperSaturationLimit=inf  LowerSaturationLimit=-inf  LinearizeAsGain=off  AntiWindupMode=none  Kb=1  TrackingMode=off  Kt=1  PParamMin=[]  PParamMax=[]  IParamMin=[]  IParamMax=[]  DParamMin=[]  DParamMax=[]  NParamMin=[]  NParamMax=[]  bParamMin=[]  bParamMax=[]  cParamMin=[]  cParamMax=[]  KbParamMin=[]  KbParamMax=[]  KtParamMin=[]  KtParamMax=[]  POutMin=[]  POutMax=[]  IOutMin=[]  IOutMax=[]  DOutMin=[]  DOutMax=[]  NOutMin=[]  NOutMax=[]  bOutMin=[]  bOutMax=[]  cOutMin=[]  cOutMax=[]  KbOutMin=[]  KbOutMax=[]  KtOutMin=[]  KtOutMax=[]  IntegratorOutMin=[]  IntegratorOutMax=[]  FilterOutMin=[]  FilterOutMax=[]  SumOutMin=[]  SumOutMax=[]  Sum1OutMin=[]  Sum1OutMax=[]  Sum2OutMin=[]  Sum2OutMax=[]  Sum3OutMin=[]  Sum3OutMax=[]  SumI1OutMin=[]  SumI1OutMax=[]  SumI2OutMin=[]  SumI2OutMax=[]  SumI3OutMin=[]  SumI3OutMax=[]  SumDOutMin=[]  SumDOutMax=[]  SaturationOutMin=[]  SaturationOutMax=[]  IntegratorContinuousStateAttributes=''  IntegratorStateMustResolveToSignalObject=off  IntegratorRTWStateStorageClass=Auto  FilterContinuousStateAttributes=''  FilterStateMustResolveToSignalObject=off  FilterRTWStateStorageClass=Auto  DifferentiatorICPrevScaledInput=0  DifferentiatorOutMin=[]  DifferentiatorOutMax=[]  FilterDiffOutCoefMin=[]  FilterDiffOutCoefMax=[]  SumDenOutMin=[]  SumDenOutMax=[]  SumNumOutMin=[]  SumNumOutMax=[]  ReciprocalOutMin=[]  ReciprocalOutMax=[]  DivideOutMin=[]  DivideOutMax=[]  TunerSelectOption=Transfer Function Based (PID Tuner App)
  cyemi_144 : DataTypeConversion  OutDataTypeStr=uint16
  cyemi_{145..155} (11 alike) : DataTypeConversion  OutDataTypeStr=double
  cfblk2 : Outport
  cfblk15 : Outport  Port=2
  cfblk16 : Outport  Port=3
  cfblk17 : Outport  Port=4
  wires:
  cfblk4/1 -> cfblk15/1
  cfblk3/1 -> cfblk17/1
  cfblk6/1 -> cfblk16/1, cyemi_153/1
  cfblk10/1 -> cfblk2/1
  cyemi_144/1 -> cfblk10/1
  cfblk14/1 -> cyemi_144/1
  cyemi_145/1 -> cfblk11/1
  cfblk9/1 -> cyemi_145/1
  cyemi_146/1 -> cfblk18/1
  cfblk11/1 -> cyemi_146/1
  cyemi_147/1 -> cfblk19/1
  cfblk7/1 -> cyemi_147/1
  cyemi_148/1 -> cfblk3/1
  cfblk12/1 -> cyemi_148/1
  cyemi_149/1 -> cfblk4/1
  cfblk8/1 -> cyemi_149/1
  cyemi_150/1 -> cfblk5/1
  cfblk19/1 -> cyemi_150/1
  cyemi_151/1 -> cfblk6/1
  cfblk13/1 -> cyemi_151/1
  cyemi_152/1 -> cfblk7/1
  cfblk5/1 -> cyemi_152/1
  cyemi_153/1 -> cfblk8/1
  cyemi_154/1 -> cfblk9/1
  cfblk1/1 -> cyemi_154/1
  cyemi_155/1 -> cfblk9/2
  cfblk18/1 -> cyemi_155/1

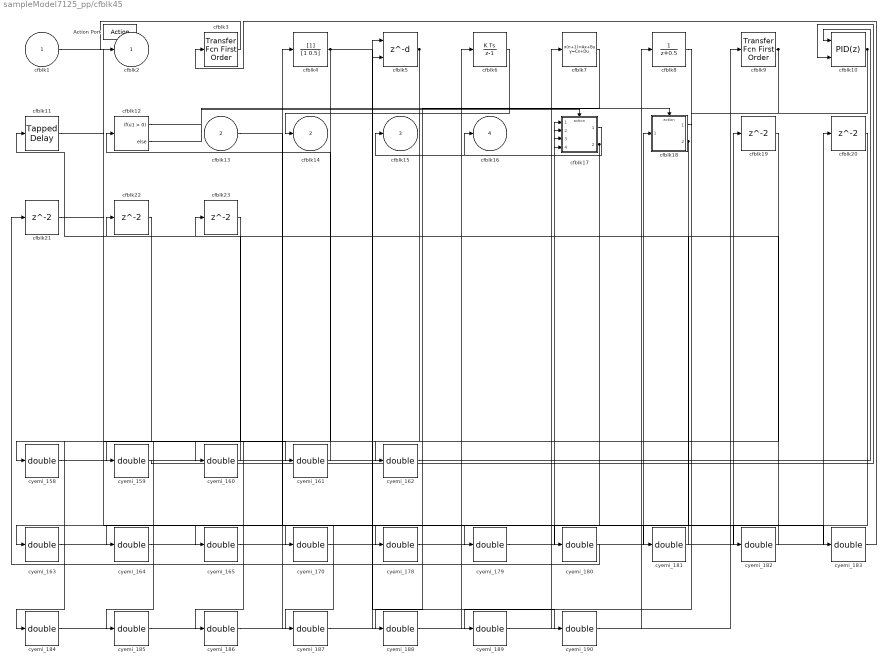
== system sampleModel7125_pp/cfblk45 ==
  cfblk1 : Inport
  cfblk13 : Inport  Port=2
  Action Port : ActionPort  ActionType=then
  cfblk10 : simulink/Continuous/PID Controller (2DOF)  Controller=PID  TimeDomain=Discrete-time  SampleTime=-1  IntegratorMethod=Forward Euler  FilterMethod=Forward Euler  Form=Parallel  UseFilter=on  ControllerParametersSource=internal  P=1  I=1  D=0  N=100  b=1  c=1  InitialConditionSource=internal  InitialConditionForIntegrator=0  InitialConditionForFilter=0  ExternalReset=none  LimitOutput=off  UpperSaturationLimit=inf  LowerSaturationLimit=-inf  LinearizeAsGain=off  AntiWindupMode=none  Kb=1  TrackingMode=off  Kt=1  PParamMin=[]  PParamMax=[]  IParamMin=[]  IParamMax=[]  DParamMin=[]  DParamMax=[]  NParamMin=[]  NParamMax=[]  bParamMin=[]  bParamMax=[]  cParamMin=[]  cParamMax=[]  KbParamMin=[]  KbParamMax=[]  KtParamMin=[]  KtParamMax=[]  POutMin=[]  POutMax=[]  IOutMin=[]  IOutMax=[]  DOutMin=[]  DOutMax=[]  NOutMin=[]  NOutMax=[]  bOutMin=[]  bOutMax=[]  cOutMin=[]  cOutMax=[]  KbOutMin=[]  KbOutMax=[]  KtOutMin=[]  KtOutMax=[]  IntegratorOutMin=[]  IntegratorOutMax=[]  FilterOutMin=[]  FilterOutMax=[]  SumOutMin=[]  SumOutMax=[]  Sum1OutMin=[]  Sum1OutMax=[]  Sum2OutMin=[]  Sum2OutMax=[]  Sum3OutMin=[]  Sum3OutMax=[]  SumI1OutMin=[]  SumI1OutMax=[]  SumI2OutMin=[]  SumI2OutMax=[]  SumI3OutMin=[]  SumI3OutMax=[]  SumDOutMin=[]  SumDOutMax=[]  SaturationOutMin=[]  SaturationOutMax=[]  IntegratorContinuousStateAttributes=''  IntegratorStateMustResolveToSignalObject=off  IntegratorRTWStateStorageClass=Auto  FilterContinuousStateAttributes=''  FilterStateMustResolveToSignalObject=off  FilterRTWStateStorageClass=Auto  DifferentiatorICPrevScaledInput=0  DifferentiatorOutMin=[]  DifferentiatorOutMax=[]  FilterDiffOutCoefMin=[]  FilterDiffOutCoefMax=[]  SumDenOutMin=[]  SumDenOutMax=[]  SumNumOutMin=[]  SumNumOutMax=[]  ReciprocalOutMin=[]  ReciprocalOutMax=[]  DivideOutMin=[]  DivideOutMax=[]  TunerSelectOption=Transfer Function Based (PID Tuner App)
  cfblk11 : simulink/Discrete/Tapped Delay  vinit=0.0  samptime=-1  NumDelays=1  DelayOrder=Oldest  includeCurrent=off
  cfblk12 : If  SampleTime=1
  cfblk17 : Subsystem  TreatAsAtomicUnit=on
  cfblk18 : Subsystem  TreatAsAtomicUnit=on
  cfblk{19..23} (5 alike) : Delay
  cfblk3 : simulink/Discrete/Transfer Fcn First Order  PoleZ=0.95  ICPrevOutput=0.0  DoSatur=off
      settings: SourceProductName=Simulink
  cfblk4 : DiscreteFilter
  cfblk5 : Delay  DelayLengthSource=Input port
      settings: InputPortMap=u0,p1
  cfblk6 : DiscreteIntegrator  SampleTime=-1  OutDataTypeStr=double  ICPrevOutput=DiscIntNeverNeededParam  ICPrevScaledInput=DiscIntNeverNeededParam
  cfblk7 : DiscreteStateSpace  SampleTime=-1
  cfblk8 : DiscreteTransferFcn
  cfblk9 : simulink/Discrete/Transfer Fcn First Order  PoleZ=0.95  ICPrevOutput=0.0  DoSatur=off
      settings: SourceProductName=Simulink
  cyemi_{158..165,170,178..190} (22 alike) : DataTypeConversion  OutDataTypeStr=double
  cfblk2 : Outport
  cfblk14 : Outport  Port=2
  cfblk15 : Outport  Port=3
  cfblk16 : Outport  Port=4
  wires:
  cfblk6/1 -> cfblk14/1
  cfblk9/1 -> cyemi_164/1, cyemi_189/1
  cfblk3/1 -> cfblk2/1
  cfblk4/1 -> cyemi_186/1, cyemi_190/1
  cfblk17/1(cfblk2) -> cfblk15/1
  cfblk10/1 -> cyemi_179/1, cyemi_180/1
  cfblk5/1 -> cyemi_158/1, cyemi_160/1
  cfblk17/2(cfblk10) -> cfblk16/1, cyemi_187/1
  cfblk18/2(cfblk9) -> cyemi_159/1, cyemi_188/1
  cfblk12/1 -> cfblk17/Action
  cfblk12/2 -> cfblk18/Action
  cyemi_158/1 -> cfblk10/1
  cyemi_159/1 -> cfblk10/2
  cyemi_160/1 -> cfblk11/1
  cyemi_161/1 -> cfblk12/1
  cfblk1/1 -> cyemi_161/1
  cyemi_162/1 -> cfblk17/1(cfblk1)
  cfblk19/1 -> cyemi_162/1
  cyemi_163/1 -> cfblk17/2(cfblk7)
  cfblk18/1(cfblk2) -> cyemi_163/1
  cyemi_164/1 -> cfblk17/3(cfblk8)
  cyemi_165/1 -> cfblk17/4(cfblk9)
  cfblk21/1 -> cyemi_165/1
  cyemi_170/1 -> cfblk18/1(cfblk1)
  cfblk20/1 -> cyemi_170/1
  cyemi_178/1 -> cfblk19/1
  cfblk7/1 -> cyemi_178/1
  cyemi_179/1 -> cfblk20/1
  cyemi_180/1 -> cfblk21/1
  cyemi_181/1 -> cfblk22/1
  cfblk8/1 -> cyemi_181/1
  cyemi_182/1 -> cfblk23/1
  cfblk11/1 -> cyemi_182/1
  cyemi_183/1 -> cfblk3/1
  cfblk13/1 -> cyemi_183/1
  cyemi_184/1 -> cfblk4/1
  cfblk22/1 -> cyemi_184/1
  cyemi_185/1 -> cfblk5/1
  cfblk23/1 -> cyemi_185/1
  cyemi_186/1 -> cfblk5/2
  cyemi_187/1 -> cfblk6/1
  cyemi_188/1 -> cfblk7/1
  cyemi_189/1 -> cfblk8/1
  cyemi_190/1 -> cfblk9/1

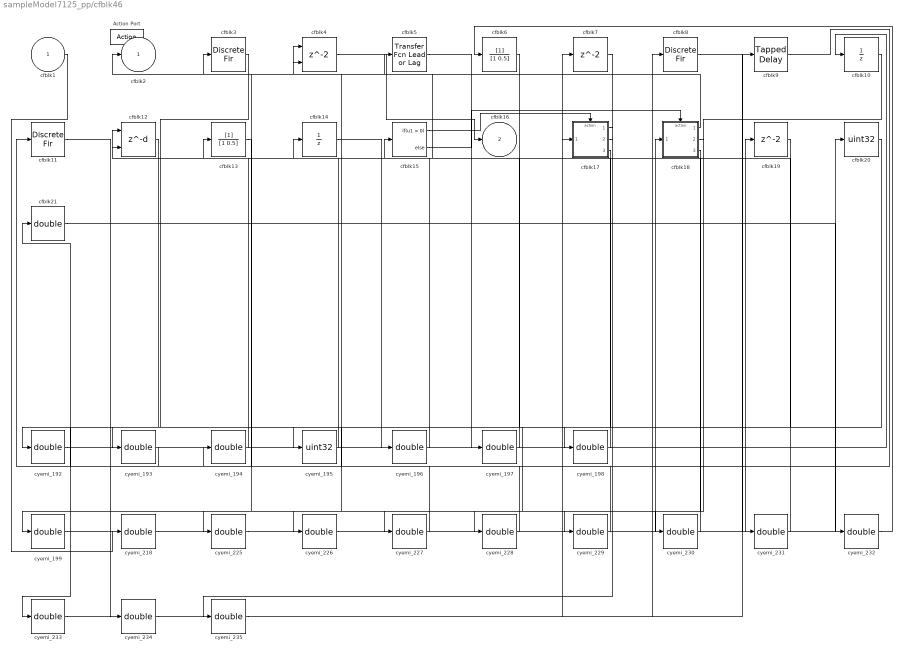
== system sampleModel7125_pp/cfblk46 ==
  cfblk1 : Inport
  Action Port : ActionPort  ActionType=else
  cfblk10 : UnitDelay  SampleTime=-1
  cfblk11 : DiscreteFir
  cfblk12 : Delay  DelayLengthSource=Input port
      settings: InputPortMap=u0,p1
  cfblk13 : DiscreteFilter
  cfblk14 : UnitDelay  SampleTime=-1
  cfblk15 : If  SampleTime=1
  cfblk17 : Subsystem  TreatAsAtomicUnit=on
  cfblk18 : Subsystem  TreatAsAtomicUnit=on
  cfblk19 : Delay
  cfblk20 : DataTypeConversion  OutDataTypeStr=uint32
  cfblk21 : DataTypeConversion  OutDataTypeStr=double
  cfblk3 : DiscreteFir
  cfblk4 : Delay  ShowEnablePort=on
      settings: InputPortMap=u0,e6
  cfblk5 : simulink/Discrete/Transfer Fcn Lead or Lag  PoleZ=0.95  ZeroZ=0.75  ICPrevOutput=0.0  ICPrevInput=0.0  DoSatur=off
      settings: SourceProductName=Simulink  SourceProductBaseCode=SL
  cfblk6 : DiscreteFilter
  cfblk7 : Delay
  cfblk8 : DiscreteFir
  cfblk9 : simulink/Discrete/Tapped Delay  vinit=0.0  samptime=-1  NumDelays=1  DelayOrder=Oldest  includeCurrent=off
  cyemi_{192..194,196..199,218,225..235} (19 alike) : DataTypeConversion  OutDataTypeStr=double
  cyemi_195 : DataTypeConversion  OutDataTypeStr=uint32
  cfblk2 : Outport
  cfblk16 : Outport  Port=2
  wires:
  cfblk18/1(cfblk2) -> cfblk2/1
  cfblk4/1 -> cfblk16/1
  cfblk15/1 -> cfblk17/Action
  cfblk15/2 -> cfblk18/Action
  cyemi_192/1 -> cfblk10/1
  cfblk17/2(cfblk15) -> cyemi_192/1
  cyemi_193/1 -> cfblk11/1
  cfblk3/1 -> cyemi_193/1
  cyemi_194/1 -> cfblk12/1
  cfblk9/1 -> cyemi_194/1
  cyemi_195/1 -> cfblk12/2
  cfblk20/1 -> cyemi_195/1
  cyemi_196/1 -> cfblk13/1
  cfblk14/1 -> cyemi_196/1
  cyemi_197/1 -> cfblk14/1
  cfblk5/1 -> cyemi_197/1
  cyemi_198/1 -> cfblk15/1
  cfblk19/1 -> cyemi_198/1
  cyemi_199/1 -> cfblk17/1(cfblk1)
  cfblk18/3(cfblk9) -> cyemi_199/1
  cyemi_218/1 -> cfblk18/1(cfblk1)
  cfblk1/1 -> cyemi_218/1
  cyemi_225/1 -> cfblk19/1
  cfblk13/1 -> cyemi_225/1
  cyemi_226/1 -> cfblk20/1
  cfblk6/1 -> cyemi_226/1
  cyemi_227/1 -> cfblk21/1
  cfblk10/1 -> cyemi_227/1
  cyemi_228/1 -> cfblk3/1
  cfblk17/3(cfblk16) -> cyemi_228/1
  cyemi_229/1 -> cfblk4/1
  cfblk7/1 -> cyemi_229/1
  cyemi_230/1 -> cfblk4/2
  cfblk18/2(cfblk8) -> cyemi_230/1
  cyemi_231/1 -> cfblk5/1
  cfblk8/1 -> cyemi_231/1
  cyemi_232/1 -> cfblk6/1
  cfblk21/1 -> cyemi_232/1
  cyemi_233/1 -> cfblk7/1
  cfblk12/1 -> cyemi_233/1
  cyemi_234/1 -> cfblk8/1
  cfblk11/1 -> cyemi_234/1
  cyemi_235/1 -> cfblk9/1
  cfblk17/1(cfblk2) -> cyemi_235/1

== system sampleModel7125_pp/cfblk47 ==
  cfblk1 : Inport
  cfblk12 : Inport  Port=2
  Action Port : ActionPort  ActionType=then
  cfblk10 : simulink/Continuous/PID Controller  Controller=PID  TimeDomain=Discrete-time  SampleTime=-1  IntegratorMethod=Forward Euler  FilterMethod=Forward Euler  Form=Parallel  UseFilter=on  ControllerParametersSource=internal  P=1  I=1  D=0  N=100  InitialConditionSource=internal  InitialConditionForIntegrator=0  InitialConditionForFilter=0  ExternalReset=none  LimitOutput=off  UpperSaturationLimit=inf  LowerSaturationLimit=-inf  LinearizeAsGain=off  AntiWindupMode=none  Kb=1  TrackingMode=off  Kt=1  PParamMin=[]  PParamMax=[]  IParamMin=[]  IParamMax=[]  DParamMin=[]  DParamMax=[]  NParamMin=[]  NParamMax=[]  KbParamMin=[]  KbParamMax=[]  KtParamMin=[]  KtParamMax=[]  POutMin=[]  POutMax=[]  IOutMin=[]  IOutMax=[]  DOutMin=[]  DOutMax=[]  NOutMin=[]  NOutMax=[]  KbOutMin=[]  KbOutMax=[]  KtOutMin=[]  KtOutMax=[]  IntegratorOutMin=[]  IntegratorOutMax=[]  FilterOutMin=[]  FilterOutMax=[]  SumOutMin=[]  SumOutMax=[]  SumI1OutMin=[]  SumI1OutMax=[]  SumI2OutMin=[]  SumI2OutMax=[]  SumI3OutMin=[]  SumI3OutMax=[]  SumDOutMin=[]  SumDOutMax=[]  SaturationOutMin=[]  SaturationOutMax=[]  IntegratorContinuousStateAttributes=''  IntegratorStateMustResolveToSignalObject=off  IntegratorRTWStateStorageClass=Auto  FilterContinuousStateAttributes=''  FilterStateMustResolveToSignalObject=off  FilterRTWStateStorageClass=Auto  DifferentiatorICPrevScaledInput=0  DifferentiatorOutMin=[]  DifferentiatorOutMax=[]  FilterDiffOutCoefMin=[]  FilterDiffOutCoefMax=[]  SumDenOutMin=[]  SumDenOutMax=[]  SumNumOutMin=[]  SumNumOutMax=[]  ReciprocalOutMin=[]  ReciprocalOutMax=[]  DivideOutMin=[]  DivideOutMax=[]  TunerSelectOption=Transfer Function Based (PID Tuner App)
  cfblk11 : DiscreteFilter
  cfblk3 : DiscreteZeroPole  Poles=[0 0.5]  Gain=1  SampleTime=-1
  cfblk4 : simulink/Discrete/Tapped Delay  vinit=0.0  samptime=-1  NumDelays=1  DelayOrder=Oldest  includeCurrent=off
  cfblk5 : simulink/Discrete/Tapped Delay  vinit=0.0  samptime=-1  NumDelays=1  DelayOrder=Oldest  includeCurrent=off
  cfblk6 : DiscreteTransferFcn
  cfblk7 : Delay  DelayLengthSource=Input port
      settings: InputPortMap=u0,p1
  cfblk8 : simulink/Discrete/Transfer Fcn First Order  PoleZ=0.95  ICPrevOutput=0.0  DoSatur=off
      settings: SourceProductName=Simulink
  cfblk9 : simulink/Discrete/Transfer Fcn First Order  PoleZ=0.95  ICPrevOutput=0.0  DoSatur=off
      settings: SourceProductName=Simulink
  cyemi_{238..247} (10 alike) : DataTypeConversion  OutDataTypeStr=double
  cfblk2 : Outport
  cfblk13 : Outport  Port=2
  wires:
  cfblk6/1 -> cfblk2/1
  cfblk11/1 -> cyemi_242/1, cyemi_245/1
  cfblk7/1 -> cfblk13/1
  cyemi_238/1 -> cfblk10/1
  cfblk5/1 -> cyemi_238/1
  cyemi_239/1 -> cfblk11/1
  cfblk8/1 -> cyemi_239/1
  cyemi_240/1 -> cfblk3/1
  cfblk10/1 -> cyemi_240/1
  cyemi_241/1 -> cfblk4/1
  cfblk12/1 -> cyemi_241/1
  cyemi_242/1 -> cfblk5/1
  cyemi_243/1 -> cfblk6/1
  cfblk4/1 -> cyemi_243/1
  cyemi_244/1 -> cfblk7/1
  cfblk3/1 -> cyemi_244/1
  cyemi_245/1 -> cfblk7/2
  cyemi_246/1 -> cfblk8/1
  cfblk9/1 -> cyemi_246/1
  cyemi_247/1 -> cfblk9/1
  cfblk1/1 -> cyemi_247/1

== system sampleModel7125_pp/cfblk48 ==
  cfblk1 : Inport
  Action Port : ActionPort  ActionType=else
  cfblk10 : Delay
  cfblk11 : Delay
  cfblk3 : Delay  ShowEnablePort=on
      settings: InputPortMap=u0,e6
  cfblk4 : DiscreteTransferFcn
  cfblk5 : DiscreteFir
  cfblk6 : If  SampleTime=1
  cfblk8 : Subsystem  TreatAsAtomicUnit=on
  cfblk9 : Subsystem  TreatAsAtomicUnit=on
  cyemi_{249..258,264..265} (12 alike) : DataTypeConversion  OutDataTypeStr=double
  cfblk2 : Outport
  cfblk7 : Outport  Port=2
  wires:
  cfblk4/1 -> cfblk7/1
  cfblk3/1 -> cfblk2/1
  cfblk5/1 -> cyemi_252/1, cyemi_257/1, cyemi_258/1
  cfblk6/1 -> cfblk8/Action
  cfblk6/2 -> cfblk9/Action
  cyemi_249/1 -> cfblk10/1
  cfblk9/1(cfblk2) -> cyemi_249/1
  cyemi_250/1 -> cfblk11/1
  cfblk9/4(cfblk15) -> cyemi_250/1
  cyemi_251/1 -> cfblk3/1
  cfblk9/3(cfblk14) -> cyemi_251/1
  cyemi_252/1 -> cfblk3/2
  cyemi_253/1 -> cfblk4/1
  cfblk9/2(cfblk13) -> cyemi_253/1
  cyemi_254/1 -> cfblk5/1
  cfblk1/1 -> cyemi_254/1
  cyemi_255/1 -> cfblk6/1
  cfblk10/1 -> cyemi_255/1
  cyemi_256/1 -> cfblk8/1(cfblk1)
  cfblk11/1 -> cyemi_256/1
  cyemi_257/1 -> cfblk8/2(cfblk7)
  cyemi_258/1 -> cfblk8/3(cfblk8)
  cyemi_264/1 -> cfblk9/1(cfblk1)
  cfblk8/1(cfblk2) -> cyemi_264/1
  cyemi_265/1 -> cfblk9/2(cfblk12)
  cfblk8/2(cfblk9) -> cyemi_265/1

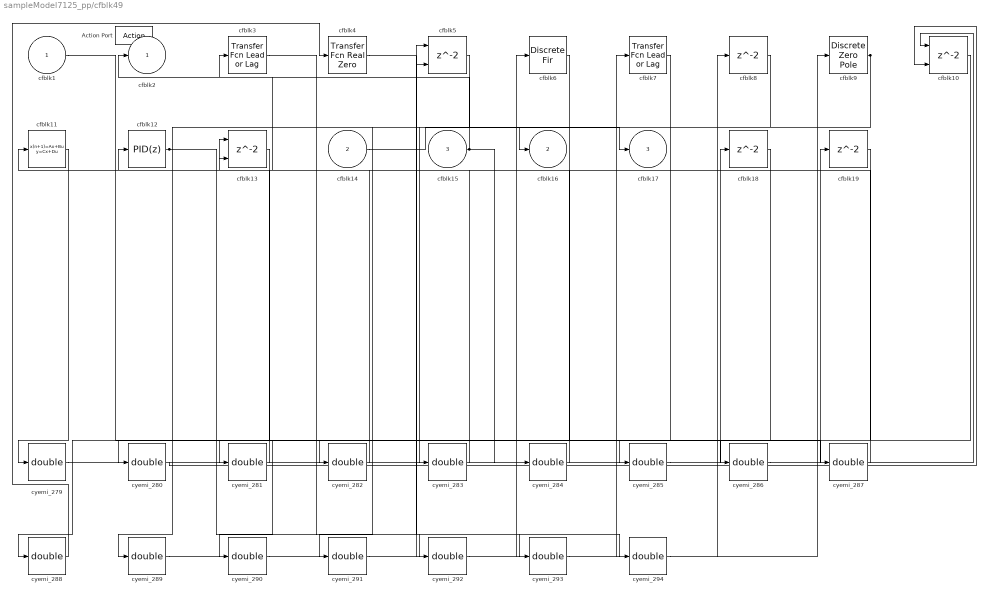
== system sampleModel7125_pp/cfblk49 ==
  cfblk1 : Inport
  cfblk14 : Inport  Port=2
  cfblk15 : Inport  Port=3
  Action Port : ActionPort  ActionType=then
  cfblk10 : Delay  ShowEnablePort=on
      settings: InputPortMap=u0,e6
  cfblk11 : DiscreteStateSpace  SampleTime=-1
  cfblk12 : simulink/Continuous/PID Controller  Controller=PID  TimeDomain=Discrete-time  SampleTime=-1  IntegratorMethod=Forward Euler  FilterMethod=Forward Euler  Form=Parallel  UseFilter=on  ControllerParametersSource=internal  P=1  I=1  D=0  N=100  InitialConditionSource=internal  InitialConditionForIntegrator=0  InitialConditionForFilter=0  ExternalReset=none  LimitOutput=off  UpperSaturationLimit=inf  LowerSaturationLimit=-inf  LinearizeAsGain=off  AntiWindupMode=none  Kb=1  TrackingMode=off  Kt=1  PParamMin=[]  PParamMax=[]  IParamMin=[]  IParamMax=[]  DParamMin=[]  DParamMax=[]  NParamMin=[]  NParamMax=[]  KbParamMin=[]  KbParamMax=[]  KtParamMin=[]  KtParamMax=[]  POutMin=[]  POutMax=[]  IOutMin=[]  IOutMax=[]  DOutMin=[]  DOutMax=[]  NOutMin=[]  NOutMax=[]  KbOutMin=[]  KbOutMax=[]  KtOutMin=[]  KtOutMax=[]  IntegratorOutMin=[]  IntegratorOutMax=[]  FilterOutMin=[]  FilterOutMax=[]  SumOutMin=[]  SumOutMax=[]  SumI1OutMin=[]  SumI1OutMax=[]  SumI2OutMin=[]  SumI2OutMax=[]  SumI3OutMin=[]  SumI3OutMax=[]  SumDOutMin=[]  SumDOutMax=[]  SaturationOutMin=[]  SaturationOutMax=[]  IntegratorContinuousStateAttributes=''  IntegratorStateMustResolveToSignalObject=off  IntegratorRTWStateStorageClass=Auto  FilterContinuousStateAttributes=''  FilterStateMustResolveToSignalObject=off  FilterRTWStateStorageClass=Auto  DifferentiatorICPrevScaledInput=0  DifferentiatorOutMin=[]  DifferentiatorOutMax=[]  FilterDiffOutCoefMin=[]  FilterDiffOutCoefMax=[]  SumDenOutMin=[]  SumDenOutMax=[]  SumNumOutMin=[]  SumNumOutMax=[]  ReciprocalOutMin=[]  ReciprocalOutMax=[]  DivideOutMin=[]  DivideOutMax=[]  TunerSelectOption=Transfer Function Based (PID Tuner App)
  cfblk13 : Delay  ShowEnablePort=on
      settings: InputPortMap=u0,e6
  cfblk18 : Delay
  cfblk19 : Delay
  cfblk3 : simulink/Discrete/Transfer Fcn Lead or Lag  PoleZ=0.95  ZeroZ=0.75  ICPrevOutput=0.0  ICPrevInput=0.0  DoSatur=off
      settings: SourceProductName=Simulink  SourceProductBaseCode=SL
  cfblk4 : simulink/Discrete/Transfer Fcn Real Zero  ZeroZ=0.75  ICPrevInput=0.0  DoSatur=off
      settings: SourceProductName=Simulink  SourceProductBaseCode=SL
  cfblk5 : Delay  ShowEnablePort=on
      settings: InputPortMap=u0,e6
  cfblk6 : DiscreteFir
  cfblk7 : simulink/Discrete/Transfer Fcn Lead or Lag  PoleZ=0.95  ZeroZ=0.75  ICPrevOutput=0.0  ICPrevInput=0.0  DoSatur=off
      settings: SourceProductName=Simulink  SourceProductBaseCode=SL
  cfblk8 : Delay
  cfblk9 : DiscreteZeroPole  Poles=[0 0.5]  Gain=1  SampleTime=-1
  cyemi_{279..294} (16 alike) : DataTypeConversion  OutDataTypeStr=double
  cfblk2 : Outport
  cfblk16 : Outport  Port=2
  cfblk17 : Outport  Port=3
  wires:
  cfblk12/1 -> cyemi_286/1, cyemi_292/1
  cfblk9/1 -> cyemi_283/1, cyemi_289/1
  cfblk15/1 -> cfblk2/1, cyemi_284/1
  cfblk14/1 -> cfblk17/1
  cfblk8/1 -> cfblk16/1
  cyemi_279/1 -> cfblk10/1
  cfblk11/1 -> cyemi_279/1
  cyemi_280/1 -> cfblk10/2
  cfblk13/1 -> cyemi_280/1
  cyemi_281/1 -> cfblk11/1
  cfblk6/1 -> cyemi_281/1
  cyemi_282/1 -> cfblk12/1
  cfblk10/1 -> cyemi_282/1
  cyemi_283/1 -> cfblk13/1
  cyemi_284/1 -> cfblk13/2
  cyemi_285/1 -> cfblk18/1
  cfblk7/1 -> cyemi_285/1
  cyemi_286/1 -> cfblk19/1
  cyemi_287/1 -> cfblk3/1
  cfblk1/1 -> cyemi_287/1
  cyemi_288/1 -> cfblk4/1
  cfblk18/1 -> cyemi_288/1
  cyemi_289/1 -> cfblk5/1
  cyemi_290/1 -> cfblk5/2
  cfblk19/1 -> cyemi_290/1
  cyemi_291/1 -> cfblk6/1
  cfblk5/1 -> cyemi_291/1
  cyemi_292/1 -> cfblk7/1
  cyemi_293/1 -> cfblk8/1
  cfblk3/1 -> cyemi_293/1
  cyemi_294/1 -> cfblk9/1
  cfblk4/1 -> cyemi_294/1

== system sampleModel7125_pp/cfblk50 ==
  cfblk1 : Inport
  cfblk12 : Inport  Port=2
  Action Port : ActionPort  ActionType=else
  cfblk10 : DiscreteZeroPole  Poles=[0 0.5]  Gain=1  SampleTime=-1
  cfblk11 : DiscreteFilter
  cfblk15 : DataTypeConversion  OutDataTypeStr=double
  cfblk16 : DataTypeConversion  OutDataTypeStr=double
  cfblk3 : DiscreteTransferFcn
  cfblk4 : DiscreteIntegrator  SampleTime=-1  OutDataTypeStr=double  ICPrevOutput=DiscIntNeverNeededParam  ICPrevScaledInput=DiscIntNeverNeededParam
  cfblk5 : simulink/Discrete/Transfer Fcn Real Zero  ZeroZ=0.75  ICPrevInput=0.0  DoSatur=off
      settings: SourceProductName=Simulink  SourceProductBaseCode=SL
  cfblk6 : DiscreteFilter
  cfblk7 : DiscreteFir
  cfblk8 : DiscreteStateSpace  SampleTime=-1
  cfblk9 : DiscreteTransferFcn
  cyemi_{299..301,303..309} (10 alike) : DataTypeConversion  OutDataTypeStr=double
  cyemi_302 : DataTypeConversion  OutDataTypeStr=uint16
  cfblk2 : Outport
  cfblk13 : Outport  Port=2
  cfblk14 : Outport  Port=3
  wires:
  cfblk8/1 -> cfblk13/1, cyemi_309/1
  cfblk1/1 -> cfblk2/1
  cfblk5/1 -> cfblk14/1
  cyemi_299/1 -> cfblk10/1
  cfblk11/1 -> cyemi_299/1
  cyemi_300/1 -> cfblk11/1
  cfblk15/1 -> cyemi_300/1
  cyemi_301/1 -> cfblk15/1
  cfblk6/1 -> cyemi_301/1
  cyemi_302/1 -> cfblk16/1
  cfblk12/1 -> cyemi_302/1
  cyemi_303/1 -> cfblk3/1
  cfblk7/1 -> cyemi_303/1
  cyemi_304/1 -> cfblk4/1
  cfblk3/1 -> cyemi_304/1
  cyemi_305/1 -> cfblk5/1
  cfblk4/1 -> cyemi_305/1
  cyemi_306/1 -> cfblk6/1
  cfblk16/1 -> cyemi_306/1
  cyemi_307/1 -> cfblk7/1
  cfblk9/1 -> cyemi_307/1
  cyemi_308/1 -> cfblk8/1
  cfblk10/1 -> cyemi_308/1
  cyemi_309/1 -> cfblk9/1
